simulink model "System_Dynamics"  (R2024b)
settings: Solver=ode45  StartTime=0.0  StopTime=60  RelTol=1e-6  AbsTol=1e-8
settings Model: Creator=LAPTOPASADI  LastModifiedBy=LAPTOPASADI

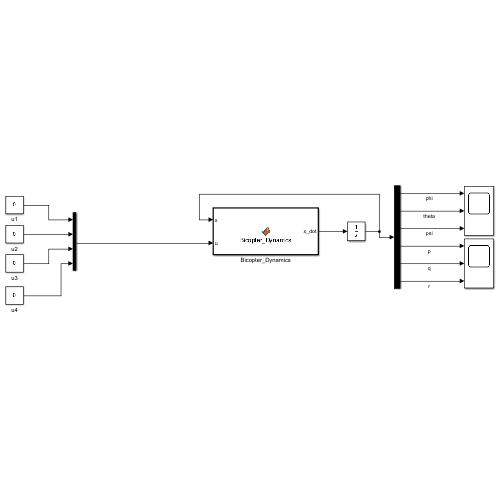
[thumbnail: Simulink's stored preview of the top-level diagram]
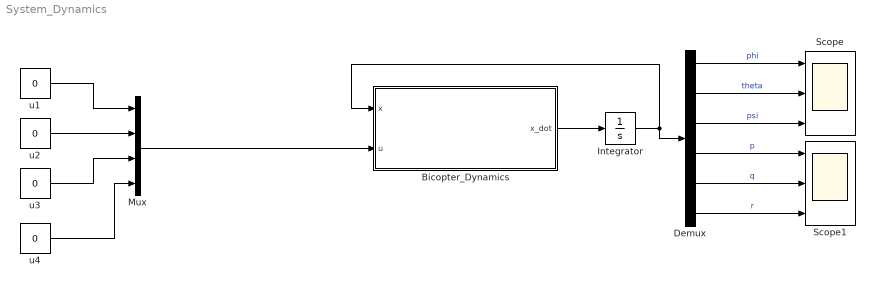
== system System_Dynamics ==
  Bicopter_Dynamics : MATLAB Function  TreatAsAtomicUnit=on
  Demux : Demux  Outputs=6
  Integrator : Integrator  InitialCondition=deg2rad([0; 0; 0; 5; 0; 0])
  Mux : Mux
  Scope : Scope  NumInputPorts=3
  Scope1 : Scope  NumInputPorts=3
  u{1..4} (4 alike) : Constant  Value=0
  wires:
  Mux/1 -> Bicopter_Dynamics/2(u)
  Bicopter_Dynamics/1(x_dot) -> Integrator/1
  Integrator/1 -> Demux/1, Bicopter_Dynamics/1(x)
  u1/1 -> Mux/1
  u2/1 -> Mux/2
  u3/1 -> Mux/3
  u4/1 -> Mux/4
  Demux/1 -> Scope/1  "phi"
  Demux/2 -> Scope/2  "theta"
  Demux/4 -> Scope1/1  "p"
  Demux/5 -> Scope1/2  "q"
  Demux/6 -> Scope1/3  "r"
  Demux/3 -> Scope/3  "psi"

== matlab function System_Dynamics/Bicopter_Dynamics ==
  data: x input; u input; x_dot output
function x_dot = Bicopter_Dynamics(x, u)
% BICOPTER_DYNAMICS
% Inputs:  x (6x1) = [phi; theta; psi; p; q; r]
%          u (4x1) = [u1; u2; u3; u4]
% Output:  x_dot (6x1) = state derivative

%% --- System Parameters ---
Ixx = 0.0043;  Iyy = 0.0142;  Izz = 0.0176;  Ixz = 0.0001;
I   = [Ixx, 0, -Ixz;
       0,   Iyy, 0;
      -Ixz, 0,   Izz];

dcg      = 0.175;
hcg      = 0.085;
d_over_b = 1.2e-6 / 3.13e-5;

B_alloc = [0,  0,    dcg,      d_over_b;
           0,  hcg,  0,        0;
           0,  0,    d_over_b, -dcg];

%% --- Extract States ---
phi   = x(1);
theta = x(2);
p     = x(4);
q     = x(5);
r     = x(6);

omega = [p; q; r];

%% --- Euler Rate Matrix J(phi, theta) ---
cth = cos(theta);
if abs(cth) < 1e-6
    cth = sign(cth + 1e-6) * 1e-6;
end
J = [1,  sin(phi)*sin(theta)/cth,  cos(phi)*sin(theta)/cth;
     0,  cos(phi),                 -sin(phi);
     0,  sin(phi)/cth,              cos(phi)/cth];

%% --- State Derivative ---
euler_dot = J * omega;                          % phi_dot, theta_dot, psi_dot
tau_gyro  = -cross(omega, I * omega);           % gyroscopic torque
omega_dot = I \ (tau_gyro + B_alloc * u);       % angular acceleration

x_dot = [euler_dot; omega_dot];                 % 6x1
end
